simulink model "TP3"  (R2023b)
settings: Solver=VariableStepAuto  StartTime=0.0  StopTime=5  RelTol=1e-3
settings Model: Creator=ousso  LastModifiedBy=ousso

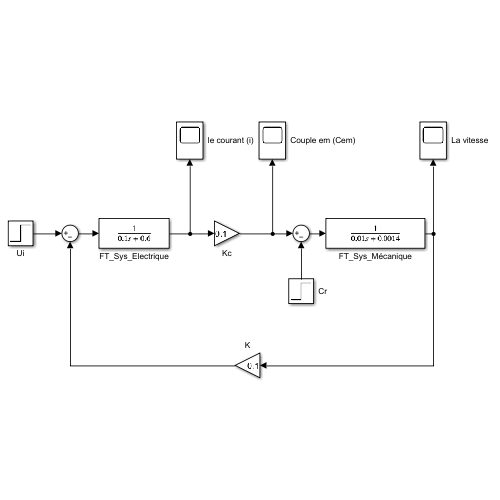
[thumbnail: Simulink's stored preview of the top-level diagram]
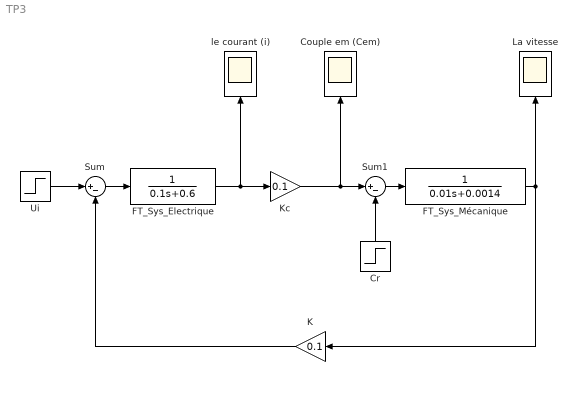
== system TP3 ==
  Couple em (Cem) : Scope
  Cr : Step  SampleTime=0
  FT_Sys_Electrique : TransferFcn  Denominator=[0.1 0.6]
  FT_Sys_Mécanique : TransferFcn  Denominator=[0.01 0.0014]
  K : Gain  Gain=0.1
  Kc : Gain  Gain=0.1
  "La vitesse " : Scope
  Sum : Sum  Inputs=|+-
  Sum1 : Sum  Inputs=|+-
  Ui : Step  Before=10  After=15  SampleTime=0
  le courant (i) : Scope
  wires:
  FT_Sys_Electrique/1 -> Kc/1, le courant (i)/1
  Ui/1 -> Sum/1
  Sum/1 -> FT_Sys_Electrique/1
  Kc/1 -> Sum1/1, Couple em (Cem)/1
  Sum1/1 -> FT_Sys_Mécanique/1
  K/1 -> Sum/2
  Cr/1 -> Sum1/2
  FT_Sys_Mécanique/1 -> K/1, "La vitesse "/1
